simulink model "untitled"  (R2017b)
settings: Solver=VariableStepAuto  StartTime=0.0  StopTime=10.0  RelTol=1e-3
libraries: simrfV2elements x1
settings Model: Creator=gzucchel  LastModifiedBy=gzucchel

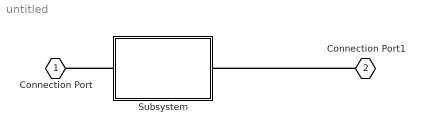
== system untitled ==
  Subsystem : Subsystem
  Connection Port : PMIOPort  Port=1  Side=Left
  Connection Port1 : PMIOPort  Port=2  Side=Left
  connections:
  Subsystem/LConn1 -- Connection Port/RConn1
  Connection Port1/RConn1 -- Subsystem/RConn1

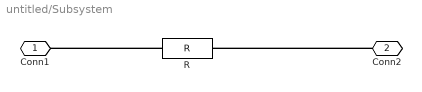
== system untitled/Subsystem ==
  R : simrfV2elements/R  classname=resistor  Resistance=50 Ohm  AddNoise=on
      settings: SourceProductName=SimRF  SourceProductBaseCode=RB
  Conn1 : PMIOPort  Port=1  Side=Left
  Conn2 : PMIOPort  Port=2  Side=Right
  connections:
  R/LConn1 -- Conn1/RConn1
  Conn2/RConn1 -- R/RConn1
